simulink model "BLDC_DTC"  (R2013a)
settings: Solver=ode45  StartTime=0.0  StopTime=10.0  RelTol=1e-3
undefined symbols (not defined in the file or in its folder): DiscIntNeverNeededParam
libraries: powerlib x8, powerlib_meascontrol x4, simulink x1
settings Model: Creator=Sony  LastModifiedBy=Sony

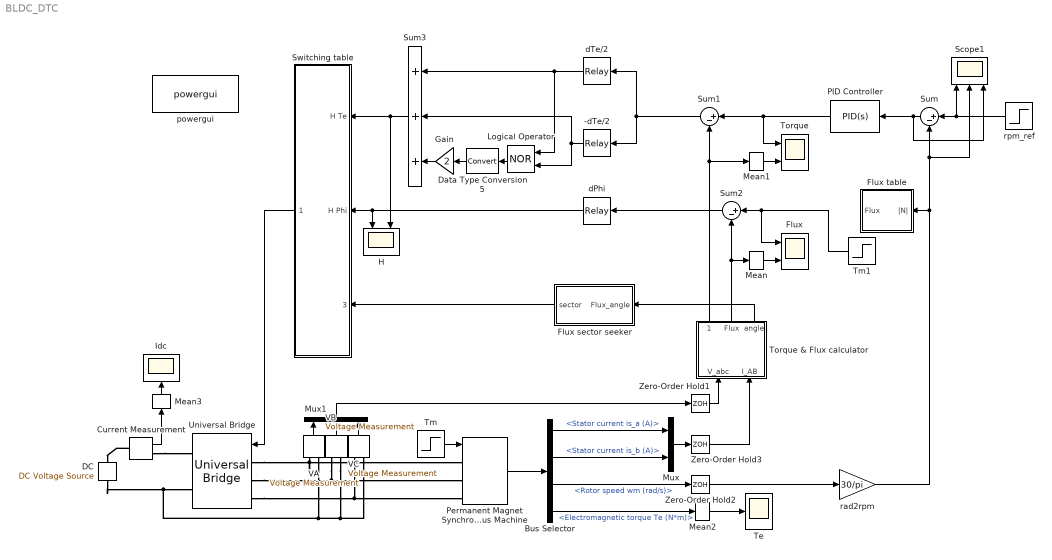
== system BLDC_DTC ==
  -dTe/2 : Relay  OnSwitchValue=0  OffSwitchValue=-1/20000  OnOutputValue=0  OffOutputValue=3
  Bus Selector : BusSelector  OutputSignals=Stator current is_a (A),Stator current is_b (A),Rotor speed wm (rad/s),Electromagnetic torque Te (N*m)
  Current Measurement : powerlib/Measurements/Current Measurement  PhasorSimulation=off  OutputType=Complex  PSBequivalent=0
  DC : powerlib/Electrical Sources/DC Voltage Source  Amplitude=48  Measurements=None
  Data Type Conversion5 : DataTypeConversion  SaturateOnIntegerOverflow=on  RndMeth=Zero
  Flux : Scope  NumInputPorts=2
      settings: YMin=0.01~0.01063  YMax=0.01~0.01081  SaveName=ScopeData2
  Flux sector seeker : Subsystem  AncestorBlock=electricdrivelib/AC drives/DTC Induction Motor Drive/DTC/Flux sector seeker
  Flux table : Subsystem  AncestorBlock=DriveInternalModels/AC drives/Speed Controller AC345/Speed Controller/Flux table  mask{bs=5000, nf=0.01}
      mask prompts: bs "Rated Speed (rpm)"; nf "Rated Stator Flux (Wb)"
      mask Display: plot([0;1800;2000;2500;3000;3500], [1;1;0.90*1;0.72*1;0.6*1;0.51*1])
  Gain : Gain  Gain=2  SaturateOnIntegerOverflow=on  OutDataTypeStr=Inherit: Same as input  ParamDataTypeStr=Inherit: Same as input
  H : Scope  NumInputPorts=2
      settings: YMin=0~0  YMax=3~4  SaveName=ScopeData6
  Idc : Scope
      settings: YMin=-200  YMax=200
  Logical Operator : Logic  Operator=NOR  AllPortsSameDT=off
  Mean{,1..3} (4 alike) : powerlib_meascontrol/Measurements/Mean  Freq=10  Vinit=0  Ts=0
  Mux : Mux  Inputs=2
  Mux1 : Mux  Inputs=3
  PID Controller : simulink/Continuous/PID Controller  Controller=PID  TimeDomain=Continuous-time  SampleTime=1  IntegratorMethod=Forward Euler  FilterMethod=Forward Euler  Form=Parallel  P=0.0001  I=0.001  D=0  N=100  InitialConditionSource=internal  InitialConditionForIntegrator=0  InitialConditionForFilter=0  ExternalReset=none  LimitOutput=on  UpperSaturationLimit=20  LowerSaturationLimit=-20  LinearizeAsGain=on  AntiWindupMode=none  Kb=1  TrackingMode=off  Kt=1  PParamMin=[]  PParamMax=[]  IParamMin=[]  IParamMax=[]  DParamMin=[]  DParamMax=[]  NParamMin=[]  NParamMax=[]  KbParamMin=[]  KbParamMax=[]  KtParamMin=[]  KtParamMax=[]  POutMin=[]  POutMax=[]  IOutMin=[]  IOutMax=[]  DOutMin=[]  DOutMax=[]  NOutMin=[]  NOutMax=[]  KbOutMin=[]  KbOutMax=[]  KtOutMin=[]  KtOutMax=[]  IntegratorOutMin=[]  IntegratorOutMax=[]  FilterOutMin=[]  FilterOutMax=[]  SumOutMin=[]  SumOutMax=[]  SumI1OutMin=[]  SumI1OutMax=[]  SumI2OutMin=[]  SumI2OutMax=[]  SumI3OutMin=[]  SumI3OutMax=[]  SumDOutMin=[]  SumDOutMax=[]  SaturationOutMin=[]  SaturationOutMax=[]  IntegratorContinuousStateAttributes=''  IntegratorStateMustResolveToSignalObject=off  IntegratorRTWStateStorageClass=Auto  FilterContinuousStateAttributes=''  FilterStateMustResolveToSignalObject=off  FilterRTWStateStorageClass=Auto
  Permanent Magnet Synchronous Machine : powerlib/Machines/Permanent Magnet Synchronous Machine  NbPhases=3  FluxDistribution=Trapezoidal  RotorType=Round  MechanicalLoad=Torque Tm  PresetModel=No  ShowDetailedParameters=on  Resistance=0.01  Inductance=1e-4  dqInductances=[8.5e-3,8.5e-3]  La=0.000835  MachineConstant=Torque Constant (N.m / A_peak)  Flux=0.0125  VoltageCst=10.472  TorqueCst=0.1  Flat=120  Mechanical=[1e-3 1e-7 4 0]  PolePairs=4  InitialConditions=[0,0, 0,0]  InitialConditions5ph=[0 0 0 0 0 0]  TsPowergui=0  TsBlock=-1  RefAngle=90 degrees behind phase A axis (modified Park)
  Scope1 : Scope  NumInputPorts=3
      settings: YMin=-5000~-5000~-1000  YMax=5000~5000~1000
  Sum : Sum  Inputs=|+-
  Sum1 : Sum  Inputs=|+-  SaturateOnIntegerOverflow=on
  Sum2 : Sum  Inputs=|+-  SaturateOnIntegerOverflow=on
  Sum3 : Sum  Inputs=+++  SaturateOnIntegerOverflow=on
  Switching table : Subsystem  AncestorBlock=electricdrivelib/AC drives/DTC Induction Motor Drive/DTC/Switching table
  Te : Scope
      settings: YMin=-4  YMax=4  SaveName=ScopeData5
  Tm : Step  Time=2  After=7  SampleTime=0
  Tm1 : Step  Time=2  Before=0.01  After=0.05  SampleTime=0
  Torque : Scope  NumInputPorts=2
      settings: YMin=-5~-5  YMax=5~5  SaveName=ScopeData3
  Torque & Flux calculator : Subsystem  AncestorBlock=electricdrivelib/AC drives/DTC Induction Motor Drive/DTC/Torque & Flux calculator  mask{Rss=0.01, P=4, Ts=1/(10000)}
  Universal Bridge : powerlib/Power Electronics/Universal Bridge  Arms=3  SnubberResistance=5000  SnubberCapacitance=1e-6  Device=MOSFET / Diodes  Ron=1e-3  Lon=0  ForwardVoltages="[  0  0  ]"  ForwardVoltage=0  GTOparameters=[ 10e-6 , 20e-6 ]  IGBTparameters=[ 1e-6 , 2e-6 ]  Measurements=None  Measurements_2=None  converterType=Rectifier
  VA : powerlib/Measurements/Voltage Measurement  PhasorSimulation=off  OutputType=Complex  PSBequivalent=0
  VB : powerlib/Measurements/Voltage Measurement  PhasorSimulation=off  OutputType=Complex  PSBequivalent=0
  VC : powerlib/Measurements/Voltage Measurement  PhasorSimulation=off  OutputType=Complex  PSBequivalent=0
  Zero-Order Hold1 : ZeroOrderHold  SampleTime=1/(10000)
  Zero-Order Hold2 : ZeroOrderHold  SampleTime=1/(10000)
  Zero-Order Hold3 : ZeroOrderHold  SampleTime=1/(10000)
  dPhi : Relay  OnSwitchValue=1/20000  OffSwitchValue=-1/20000  OffOutputValue=2
  dTe/2 : Relay  OnSwitchValue=1/20000  OffSwitchValue=0
  powergui : powerlib/powergui  Priority=2  SimulationMode=Discrete  SolverType=Backward Euler  SampleTime=1e-5  frequency=60  SPID=off  DisableSnubberDevices=off  DisableRonSwitches=off  DisableVfSwitches=off  SwTol=0  Interpol=off  DisplayEquations=off  frequencyindice=0  Pbase=100e6  ErrMax=1e-4  Iterations=50  UnitsV=kV  UnitsW=MW  FunctionMessages=off  echomessages=off  HookPort=off  EnableUseOfTLC=off  x0status=blocks  RestoreLinks=warning  ResistiveCurrentMeasurement=off  Frange=[0:2:500]  Ylog=off  Xlog=on  ShowGrid=off  save=off  variable=ZData  ZoomFFT=on  StartTime=0.0  cycles=1  DisplayStyle=1  fundamental=60  FreqAxis=off  MaxFrequency=1000  frequencyindicesteady=1  RmsSteady=1  display=off  Ts=0  methode=off
  rad2rpm : Gain  Gain=30/pi
  rpm_ref : Step  Time=5  Before=4000  After=4000  SampleTime=0
  wires:
  Bus Selector/1 -> Mux/1  "<Stator current is_a (A)>"
  Permanent Magnet Synchronous Machine/1 -> Bus Selector/1
  Bus Selector/2 -> Mux/2  "<Stator current is_b (A)>"
  Bus Selector/3 -> Zero-Order Hold2/1  "<Rotor speed wm (rad/s)>"
  Sum/1 -> Scope1/3, PID Controller/1
  rpm_ref/1 -> Scope1/1, Sum/1
  Tm/1 -> Permanent Magnet Synchronous Machine/1
  Torque & Flux calculator/1(Torque) -> Mean1/1, Sum1/2
  Torque & Flux calculator/2(Flux) -> Mean/1, Sum2/2
  Torque & Flux calculator/3(angle) -> Flux sector seeker/1(Flux_angle)
  Flux sector seeker/1(sector) -> Switching table/3(Sector)
  dPhi/1 -> H/1, Switching table/2(H Phi)
  Switching table/1(Gates) -> Universal Bridge/1
  Mux/1 -> Zero-Order Hold3/1
  VA/1 -> Mux1/1
  VB/1 -> Mux1/2
  VC/1 -> Mux1/3
  Mux1/1 -> Zero-Order Hold1/1
  Tm1/1 -> Flux/1, Sum2/1
  Sum3/1 -> Switching table/1(H Te), H/2
  Data Type Conversion5/1 -> Gain/1
  Gain/1 -> Sum3/3
  Logical Operator/1 -> Data Type Conversion5/1
  Sum1/1 -> -dTe/2/1, dTe/2/1
  dTe/2/1 -> Logical Operator/1, Sum3/1
  -dTe/2/1 -> Logical Operator/2, Sum3/2
  Sum2/1 -> dPhi/1
  Zero-Order Hold1/1 -> Torque & Flux calculator/1(V_abc)
  Zero-Order Hold3/1 -> Torque & Flux calculator/2(I_AB)
  Zero-Order Hold2/1 -> rad2rpm/1
  Current Measurement/1 -> Mean3/1
  Mean3/1 -> Idc/1
  rad2rpm/1 -> Flux table/1(|N|), Sum/2, Scope1/2
  PID Controller/1 -> Sum1/1, Torque/1
  Mean2/1 -> Te/1
  Bus Selector/4 -> Mean2/1  "<Electromagnetic torque Te (N*m)>"
  Mean1/1 -> Torque/2
  Mean/1 -> Flux/2
  connections:
  Universal Bridge/LConn1 -- VA/LConn1 -- Permanent Magnet Synchronous Machine/LConn1
  DC/LConn1 -- VB/LConn2 -- VC/LConn2 -- VA/LConn2 -- Universal Bridge/RConn2
  Universal Bridge/LConn2 -- VB/LConn1 -- Permanent Magnet Synchronous Machine/LConn2
  Universal Bridge/LConn3 -- VC/LConn1 -- Permanent Magnet Synchronous Machine/LConn3
  Current Measurement/RConn1 -- Universal Bridge/RConn1
  Current Measurement/LConn1 -- DC/RConn1

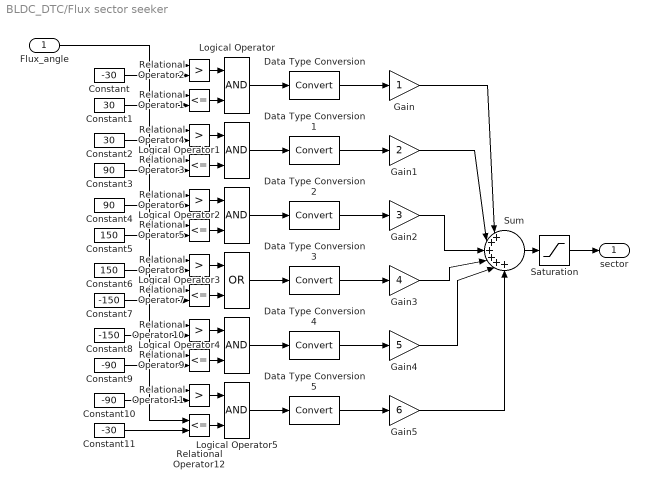
== system BLDC_DTC/Flux sector seeker ==
  Flux_angle : Inport
  Constant : Constant  Value=-30
  Constant1 : Constant  Value=30
  Constant10 : Constant  Value=-90
  Constant11 : Constant  Value=-30
  Constant2 : Constant  Value=30
  Constant3 : Constant  Value=90
  Constant4 : Constant  Value=90
  Constant5 : Constant  Value=150
  Constant6 : Constant  Value=150
  Constant7 : Constant  Value=-150
  Constant8 : Constant  Value=-150
  Constant9 : Constant  Value=-90
  Data Type Conversion{,1..5} (6 alike) : DataTypeConversion  SaturateOnIntegerOverflow=on  RndMeth=Zero
  Gain : Gain  SaturateOnIntegerOverflow=on  OutDataTypeStr=Inherit: Same as input  ParamDataTypeStr=Inherit: Same as input
  Gain1 : Gain  Gain=2  SaturateOnIntegerOverflow=on  OutDataTypeStr=Inherit: Same as input  ParamDataTypeStr=Inherit: Same as input
  Gain2 : Gain  Gain=3  SaturateOnIntegerOverflow=on  OutDataTypeStr=Inherit: Same as input  ParamDataTypeStr=Inherit: Same as input
  Gain3 : Gain  Gain=4  SaturateOnIntegerOverflow=on  OutDataTypeStr=Inherit: Same as input  ParamDataTypeStr=Inherit: Same as input
  Gain4 : Gain  Gain=5  SaturateOnIntegerOverflow=on  OutDataTypeStr=Inherit: Same as input  ParamDataTypeStr=Inherit: Same as input
  Gain5 : Gain  Gain=6  SaturateOnIntegerOverflow=on  OutDataTypeStr=Inherit: Same as input  ParamDataTypeStr=Inherit: Same as input
  Logical Operator{,1..2,4..5} (5 alike) : Logic
  Logical Operator3 : Logic  Operator=OR
  Relational Operator{1,3,5,7,9,12} (6 alike) : RelationalOperator  Operator=<=  InputSameDT=on
  Relational Operator{2,4,6,8,10..11} (6 alike) : RelationalOperator  Operator=>  InputSameDT=on
  Saturation : Saturate  UpperLimit=6  LowerLimit=1
  Sum : Sum  Inputs=|++++++  SaturateOnIntegerOverflow=on  InputSameDT=on  OutDataTypeStr=Inherit: Same as first input
  sector : Outport
  wires:
  Data Type Conversion5/1 -> Gain5/1
  Data Type Conversion4/1 -> Gain4/1
  Data Type Conversion3/1 -> Gain3/1
  Data Type Conversion2/1 -> Gain2/1
  Data Type Conversion1/1 -> Gain1/1
  Data Type Conversion/1 -> Gain/1
  Saturation/1 -> sector/1
  Sum/1 -> Saturation/1
  Gain5/1 -> Sum/6
  Gain4/1 -> Sum/5
  Gain3/1 -> Sum/4
  Gain2/1 -> Sum/3
  Gain1/1 -> Sum/2
  Gain/1 -> Sum/1
  Constant11/1 -> Relational Operator12/2
  Constant10/1 -> Relational Operator11/2
  Logical Operator5/1 -> Data Type Conversion5/1
  Relational Operator12/1 -> Logical Operator5/2
  Relational Operator11/1 -> Logical Operator5/1
  Constant9/1 -> Relational Operator9/2
  Constant8/1 -> Relational Operator10/2
  Logical Operator4/1 -> Data Type Conversion4/1
  Relational Operator9/1 -> Logical Operator4/2
  Relational Operator10/1 -> Logical Operator4/1
  Constant7/1 -> Relational Operator7/2
  Constant6/1 -> Relational Operator8/2
  Logical Operator3/1 -> Data Type Conversion3/1
  Relational Operator7/1 -> Logical Operator3/2
  Relational Operator8/1 -> Logical Operator3/1
  Constant5/1 -> Relational Operator5/2
  Constant4/1 -> Relational Operator6/2
  Logical Operator2/1 -> Data Type Conversion2/1
  Relational Operator5/1 -> Logical Operator2/2
  Relational Operator6/1 -> Logical Operator2/1
  Constant3/1 -> Relational Operator3/2
  Constant2/1 -> Relational Operator4/2
  Logical Operator1/1 -> Data Type Conversion1/1
  Relational Operator3/1 -> Logical Operator1/2
  Relational Operator4/1 -> Logical Operator1/1
  Constant1/1 -> Relational Operator1/2
  Constant/1 -> Relational Operator2/2
  Flux_angle/1 -> Relational Operator12/1, Relational Operator11/1, Relational Operator9/1, Relational Operator10/1, Relational Operator7/1, Relational Operator8/1, Relational Operator5/1, Relational Operator6/1, Relational Operator3/1, Relational Operator4/1, Relational Operator1/1, Relational Operator2/1
  Logical Operator/1 -> Data Type Conversion/1
  Relational Operator1/1 -> Logical Operator/2
  Relational Operator2/1 -> Logical Operator/1

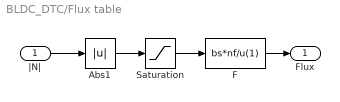
== system BLDC_DTC/Flux table ==
  |N| : Inport
  Abs1 : Abs  SaturateOnIntegerOverflow=on
  F : Fcn  Expr=bs*nf/u(1)
  Saturation : Saturate  UpperLimit=inf  LowerLimit=bs
  Flux : Outport
  wires:
  Abs1/1 -> Saturation/1
  F/1 -> Flux/1
  |N|/1 -> Abs1/1
  Saturation/1 -> F/1

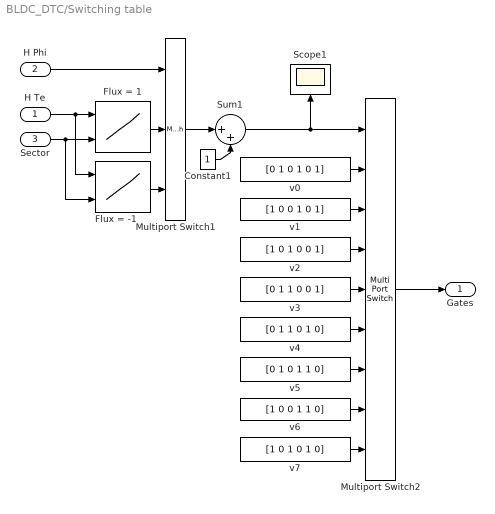
== system BLDC_DTC/Switching table ==
  H Te : Inport
  H Phi : Inport  Port=2
  Sector : Inport  Port=3
  Constant1 : Constant
  Flux = -1 : Lookup2D  RowIndex=[1;2;3]  ColumnIndex=[1;2;3;4;5;6]  Table=[3 4 5 6 1 2;7 0 7 0 7 0;5 6 1 2 3 4]  SaturateOnIntegerOverflow=on
  Flux = 1 : Lookup2D  RowIndex=[1;2;3]  ColumnIndex=[1;2;3;4;5;6]  Table=[2 3 4 5 6 1;0 7 0 7 0 7;6 1 2 3 4 5]  SaturateOnIntegerOverflow=on
  Multiport Switch1 : MultiPortSwitch  Inputs=2  SaturateOnIntegerOverflow=on
  Multiport Switch2 : MultiPortSwitch  Inputs=8  SaturateOnIntegerOverflow=on
  Scope1 : Scope
      settings: YMin=-1  YMax=10  SaveName=ScopeData4
  Sum1 : Sum  Inputs=|++  SaturateOnIntegerOverflow=on
  v0 : Constant  Value=[0 1 0 1 0 1]
  v1 : Constant  Value=[1 0 0 1 0 1]
  v2 : Constant  Value=[1 0 1 0 0 1]
  v3 : Constant  Value=[0 1 1 0 0 1]
  v4 : Constant  Value=[0 1 1 0 1 0]
  v5 : Constant  Value=[0 1 0 1 1 0]
  v6 : Constant  Value=[1 0 0 1 1 0]
  v7 : Constant  Value=[1 0 1 0 1 0]
  Gates : Outport
  wires:
  Multiport Switch2/1 -> Gates/1
  v5/1 -> Multiport Switch2/7
  v3/1 -> Multiport Switch2/5
  v6/1 -> Multiport Switch2/8
  v2/1 -> Multiport Switch2/4
  Multiport Switch1/1 -> Sum1/1
  Sum1/1 -> Scope1/1, Multiport Switch2/1
  Constant1/1 -> Sum1/2
  Flux = -1/1 -> Multiport Switch1/3
  Flux = 1/1 -> Multiport Switch1/2
  H Phi/1 -> Multiport Switch1/1
  Sector/1 -> Flux = 1/2, Flux = -1/2
  v7/1 -> Multiport Switch2/9
  v4/1 -> Multiport Switch2/6
  v1/1 -> Multiport Switch2/3
  v0/1 -> Multiport Switch2/2
  H Te/1 -> Flux = 1/1, Flux = -1/1

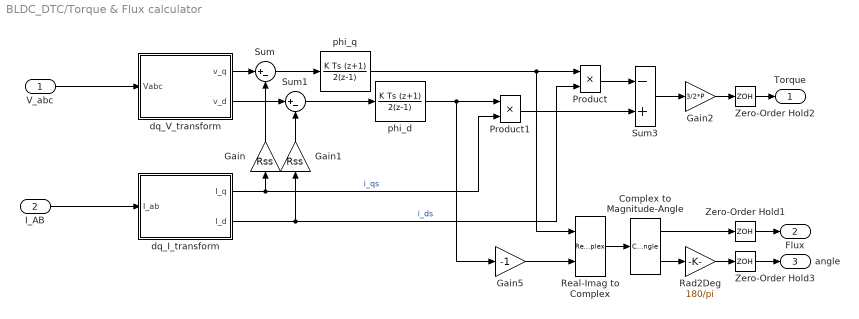
== system BLDC_DTC/Torque & Flux calculator ==
  V_abc : Inport
  I_AB : Inport  Port=2
  Complex to Magnitude-Angle : ComplexToMagnitudeAngle
  Gain : Gain  Gain=Rss  SaturateOnIntegerOverflow=on  OutDataTypeStr=Inherit: Same as input  ParamDataTypeStr=Inherit: Same as input
  Gain1 : Gain  Gain=Rss  SaturateOnIntegerOverflow=on  OutDataTypeStr=Inherit: Same as input  ParamDataTypeStr=Inherit: Same as input
  Gain2 : Gain  Gain=3/2*P  SaturateOnIntegerOverflow=on  OutDataTypeStr=Inherit: Same as input  ParamDataTypeStr=Inherit: Same as input
  Gain5 : Gain  Gain=-1  SaturateOnIntegerOverflow=on  OutDataTypeStr=Inherit: Same as input  ParamDataTypeStr=Inherit: Same as input
  Product : Product  SaturateOnIntegerOverflow=on  OutDataTypeStr=Inherit: Same as first input
  Product1 : Product  SaturateOnIntegerOverflow=on  OutDataTypeStr=Inherit: Same as first input
  Rad2Deg : Gain  Gain=180/pi  SaturateOnIntegerOverflow=on  OutDataTypeStr=Inherit: Same as input  ParamDataTypeStr=Inherit: Same as input
  Real-Imag to Complex : RealImagToComplex
  Sum : Sum  Inputs=|+-  SaturateOnIntegerOverflow=on
  Sum1 : Sum  Inputs=|+-  SaturateOnIntegerOverflow=on
  Sum3 : Sum  Inputs=-+  SaturateOnIntegerOverflow=on
  Zero-Order Hold1 : ZeroOrderHold  SampleTime=Ts
  Zero-Order Hold2 : ZeroOrderHold  SampleTime=Ts
  Zero-Order Hold3 : ZeroOrderHold  SampleTime=Ts
  dq_I_transform : Subsystem
  dq_V_transform : Subsystem
  phi_d : DiscreteIntegrator  IntegratorMethod=Integration: Trapezoidal  SampleTime=Ts  ICPrevOutput=DiscIntNeverNeededParam  ICPrevScaledInput=DiscIntNeverNeededParam
  phi_q : DiscreteIntegrator  IntegratorMethod=Integration: Trapezoidal  SampleTime=Ts  ICPrevOutput=DiscIntNeverNeededParam  ICPrevScaledInput=DiscIntNeverNeededParam
  Torque : Outport
  Flux : Outport  Port=2
  angle : Outport  Port=3
  wires:
  Zero-Order Hold3/1 -> angle/1
  Zero-Order Hold1/1 -> Flux/1
  Zero-Order Hold2/1 -> Torque/1
  Product1/1 -> Sum3/2
  Gain5/1 -> Real-Imag to Complex/2
  Rad2Deg/1 -> Zero-Order Hold3/1
  Complex to Magnitude-Angle/2 -> Rad2Deg/1
  Complex to Magnitude-Angle/1 -> Zero-Order Hold1/1
  Real-Imag to Complex/1 -> Complex to Magnitude-Angle/1
  I_AB/1 -> dq_I_transform/1(I_ab)
  V_abc/1 -> dq_V_transform/1(Vabc)
  dq_V_transform/1(v_q) -> Sum/1
  dq_I_transform/1(I_q) -> Gain/1, Product1/2  "i_qs"
  Gain/1 -> Sum/2
  Sum/1 -> phi_q/1
  dq_V_transform/2(v_d) -> Sum1/1
  Gain1/1 -> Sum1/2
  dq_I_transform/2(I_d) -> Product/2, Gain1/1  "i_ds"
  Sum1/1 -> phi_d/1
  phi_q/1 -> Real-Imag to Complex/1, Product/1
  phi_d/1 -> Product1/1, Gain5/1
  Product/1 -> Sum3/1
  Sum3/1 -> Gain2/1
  Gain2/1 -> Zero-Order Hold2/1

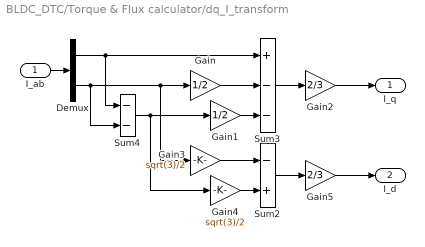
== system BLDC_DTC/Torque & Flux calculator/dq_I_transform ==
  I_ab : Inport
  Demux : Demux  Outputs=2
  Gain : Gain  Gain=1/2  SaturateOnIntegerOverflow=on  OutDataTypeStr=Inherit: Same as input  ParamDataTypeStr=Inherit: Same as input
  Gain1 : Gain  Gain=1/2  SaturateOnIntegerOverflow=on  OutDataTypeStr=Inherit: Same as input  ParamDataTypeStr=Inherit: Same as input
  Gain2 : Gain  Gain=2/3  SaturateOnIntegerOverflow=on  OutDataTypeStr=Inherit: Same as input  ParamDataTypeStr=Inherit: Same as input
  Gain3 : Gain  Gain=sqrt(3)/2  SaturateOnIntegerOverflow=on  OutDataTypeStr=Inherit: Same as input  ParamDataTypeStr=Inherit: Same as input
  Gain4 : Gain  Gain=sqrt(3)/2  SaturateOnIntegerOverflow=on  OutDataTypeStr=Inherit: Same as input  ParamDataTypeStr=Inherit: Same as input
  Gain5 : Gain  Gain=2/3  SaturateOnIntegerOverflow=on  OutDataTypeStr=Inherit: Same as input  ParamDataTypeStr=Inherit: Same as input
  Sum2 : Sum  Inputs=-+  SaturateOnIntegerOverflow=on  InputSameDT=on  OutDataTypeStr=Inherit: Same as first input
  Sum3 : Sum  Inputs=+--  SaturateOnIntegerOverflow=on  InputSameDT=on  OutDataTypeStr=Inherit: Same as first input
  Sum4 : Sum  Inputs=--  SaturateOnIntegerOverflow=on  InputSameDT=on  OutDataTypeStr=Inherit: Same as first input
  I_q : Outport
  I_d : Outport  Port=2
  wires:
  Sum2/1 -> Gain5/1
  Gain4/1 -> Sum2/2
  Gain3/1 -> Sum2/1
  Sum3/1 -> Gain2/1
  Sum4/1 -> Gain4/1, Gain1/1
  Gain/1 -> Sum3/2
  Gain1/1 -> Sum3/3
  Demux/2 -> Sum4/2, Gain/1, Gain3/1
  Demux/1 -> Sum4/1, Sum3/1
  I_ab/1 -> Demux/1
  Gain5/1 -> I_d/1
  Gain2/1 -> I_q/1

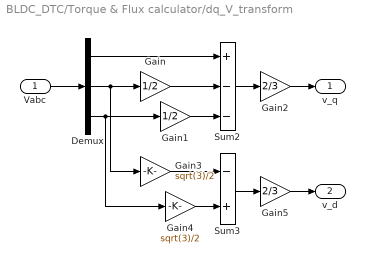
== system BLDC_DTC/Torque & Flux calculator/dq_V_transform ==
  Vabc : Inport
  Demux : Demux  Outputs=3
  Gain : Gain  Gain=1/2  SaturateOnIntegerOverflow=on  OutDataTypeStr=Inherit: Same as input  ParamDataTypeStr=Inherit: Same as input
  Gain1 : Gain  Gain=1/2  SaturateOnIntegerOverflow=on  OutDataTypeStr=Inherit: Same as input  ParamDataTypeStr=Inherit: Same as input
  Gain2 : Gain  Gain=2/3  SaturateOnIntegerOverflow=on  OutDataTypeStr=Inherit: Same as input  ParamDataTypeStr=Inherit: Same as input
  Gain3 : Gain  Gain=sqrt(3)/2  SaturateOnIntegerOverflow=on  OutDataTypeStr=Inherit: Same as input  ParamDataTypeStr=Inherit: Same as input
  Gain4 : Gain  Gain=sqrt(3)/2  SaturateOnIntegerOverflow=on  OutDataTypeStr=Inherit: Same as input  ParamDataTypeStr=Inherit: Same as input
  Gain5 : Gain  Gain=2/3  SaturateOnIntegerOverflow=on  OutDataTypeStr=Inherit: Same as input  ParamDataTypeStr=Inherit: Same as input
  Sum2 : Sum  Inputs=+--  SaturateOnIntegerOverflow=on  InputSameDT=on  OutDataTypeStr=Inherit: Same as first input
  Sum3 : Sum  Inputs=-+  SaturateOnIntegerOverflow=on  InputSameDT=on  OutDataTypeStr=Inherit: Same as first input
  v_q : Outport
  v_d : Outport  Port=2
  wires:
  Sum3/1 -> Gain5/1
  Gain4/1 -> Sum3/2
  Gain3/1 -> Sum3/1
  Gain2/1 -> v_q/1
  Gain1/1 -> Sum2/3
  Gain/1 -> Sum2/2
  Demux/1 -> Sum2/1
  Sum2/1 -> Gain2/1
  Gain5/1 -> v_d/1
  Vabc/1 -> Demux/1
  Demux/2 -> Gain/1, Gain3/1
  Demux/3 -> Gain1/1, Gain4/1
